simulink model "ThurstCalculation_Part2"  (R2017b)
settings: Solver=ode2  StartTime=0.0  StopTime=inf  FixedStep=1/100  RelTol=1e-3  EnableMultiTasking=on
libraries: aerolibatmos2 x1, aerolibconvert2 x1
settings Model: Creator=dsde009  LastModifiedBy=Danyck
settings SolverCC: AlgebraicLoopSolver=LineSearch
settings DataIOCC: LimitDataPoints=on  SaveFormat=Array  SignalLoggingSaveFormat=ModelDataLogs  SignalLoggingName=SPE_DataLog
settings OptimizationCC: ExpressionDepthLimit=2147483647  InitFltsAndDblsToZero=on  LifeSpan=inf
settings DebuggingCC: ReadBeforeWriteMsg=DisableAll  WriteAfterWriteMsg=DisableAll  WriteAfterReadMsg=DisableAll  AlgebraicLoopMsg=none  SaveWithDisabledLinksMsg=none  UnderspecifiedInitializationDetection=Classic  MergeDetectMultiDrivingBlocksExec=none  MultiTaskDSMMsg=warning  MultiTaskCondExecSysMsg=none  ParameterPrecisionLossMsg=none  StateNameClashWarn=warning  SFUnexpectedBacktrackingDiag=warning  SFNoUnconditionalDefaultTransitionDiag=warning  SFExecutionAtInitializationDiag=none
settings HardwareCC: ProdBitPerPointer=32  ProdBitPerSizeT=32  ProdBitPerPtrDiffT=32  ProdLargestAtomicFloat=None  ProdIntDivRoundTo=Undefined  ProdEndianess=Unspecified  ProdWordSize=32  ProdHWDeviceType=32-bit Generic
settings ModelReferenceCC: UpdateModelReferenceTargets=IfOutOfDate  PropagateSignalLabelsOutOfModel=off
settings SFSimCC: SFSimEcho=off
settings CodeAppCC: StateflowObjectComments=on
settings GRTTargetCC: TargetLangStandard=C89/C90 (ANSI)  GeneratePreprocessorConditionals=Disable all  CombineOutputUpdateFcns=off  GRTInterface=on
settings ConfigComp: CovMetricSettings=dw  CovHtmlReporting=on  CovSaveCumulativeToWorkspaceVar=on  CovSaveSingleToWorkspaceVar=on  CovExternalEMLEnable=off  CovSFcnEnable=off

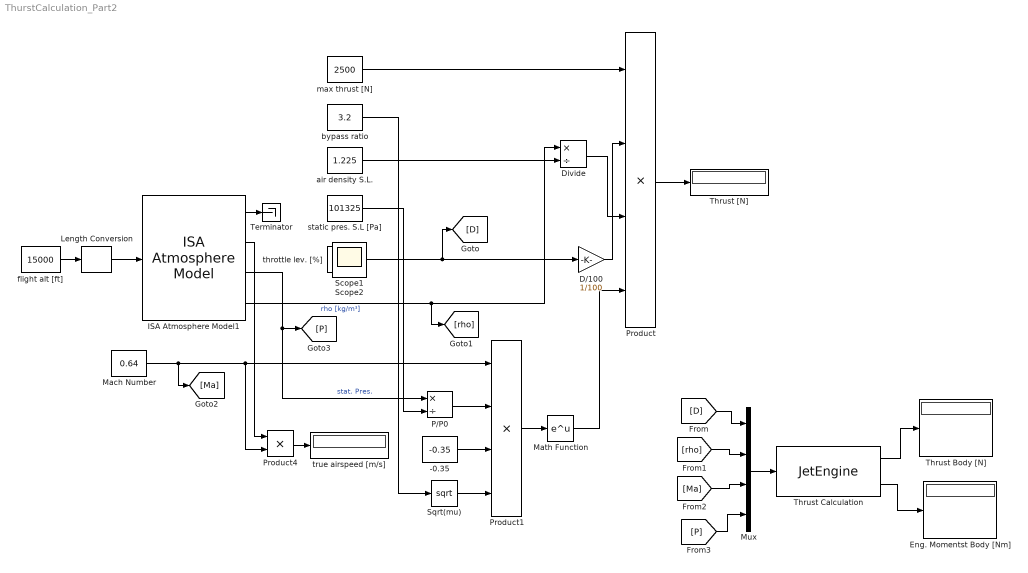
== system ThurstCalculation_Part2 ==
  -0.35 : Constant  Value=-0.35
  D/100 : Gain  Gain=1/100
  Divide : Product  Inputs=*/
  Eng. Momentst Body [Nm] : Display
  ISA Atmosphere Model1 : aerolibatmos2/ISA Atmosphere Model  custom=off  g=9.80665  gamma=1.4  R=287.0531  L=0.0065  h_trop=11000  h_strat=20000  rho0=1.225  P0=101325  T0=288.15  h0=0
      settings: SourceProductName=Aerospace Blockset
  Length Conversion : aerolibconvert2/Length Conversion  IU=ft  OU=m
  Mach Number : Constant  Value=0.64
  Math Function : Math  SaturateOnIntegerOverflow=on
  Mux : Mux
  P/P0 : Product  Inputs=*/
  Product : Product  Inputs=4
  Product1 : Product  Inputs=4
  Product4 : Product
  Sqrt(mu) : Sqrt  SaturateOnIntegerOverflow=on
  Terminator : Terminator
  Thrust Body [N] : Display
  Thrust Calculation : M-S-Function  FunctionName=JetEngine  Parameters=0
  Thrust [N] : Display
  air density S.L. : Constant  Value=1.225
  bypass ratio : Constant  Value=3.2
  flight alt [ft] : Constant  Value=15000
  max thrust [N] : Constant  Value=2500
  static pres. S.L [Pa] : Constant  Value=101325
  throttle lev. [%] : Constant  Value=85
  true airspeed [m/s] : Display
  Scope1 : Scope
  Scope2 : Scope
  wires:
  Length Conversion/1 -> ISA Atmosphere Model1/1
  max thrust [N]/1 -> Product/1
  throttle lev. [%]/1 -> [D], D/100/1
  D/100/1 -> Product/2
  air density S.L./1 -> Divide/2
  ISA Atmosphere Model1/4 -> [rho], Divide/1  "rho [kg/m³]"
  Divide/1 -> Product/3
  ISA Atmosphere Model1/3 -> [P], P/P0/1  "stat. Pres."
  static pres. S.L [Pa]/1 -> P/P0/2
  P/P0/1 -> Product1/2
  Mach Number/1 -> [Ma], Product4/2, Product1/1
  -0.35/1 -> Product1/3
  bypass ratio/1 -> Sqrt(mu)/1
  Sqrt(mu)/1 -> Product1/4
  Product1/1 -> Math Function/1
  Math Function/1 -> Product/4
  Product/1 -> Thrust [N]/1
  flight alt [ft]/1 -> Length Conversion/1
  ISA Atmosphere Model1/2 -> Product4/1
  Product4/1 -> true airspeed [m/s]/1
  ISA Atmosphere Model1/1 -> Terminator/1
  Thrust Calculation/1 -> Thrust Body [N]/1
  Thrust Calculation/2 -> Eng. Momentst Body [Nm]/1
  Mux/1 -> Thrust Calculation/1
  [P] -> Mux/4
  [Ma] -> Mux/3
  [rho] -> Mux/2
  [D] -> Mux/1
